simulink model "test_kalman_filter"  (R2020a)
settings: Solver=FixedStepAuto  StartTime=0.0  StopTime=85  RelTol=1e-3
values from neighbouring files (symbols this model uses):
  dt = 1/100    (= 0.01)    [load_tune.m]
  P0 = deg2rad(1)*eye(3,3)    [load_tune.m]
  Q = diag([a*pqr_dot_covar(1)*a /4, a*pqr_dot_covar(2)*a/4, a*pqr_dot_covar(3)*a/4])    [load_tune.m]
  R = diag([0.0155^2, 0.0124^2, 0.0147^2])    [load_tune.m]
  x0 = [0;0;0]    [load_tune.m]
undefined symbols (not defined in the file or in its folder): sim_data
libraries: myLib x3, simulink_extras x3, simulink x2, sharedtransform x1
settings Model: Creator=Test  LastModifiedBy=Jason
settings DataIOCC: ReturnWorkspaceOutputs=off
settings DebuggingCC: ArithmeticOperatorsInVariantConditions=warning
settings SFSimCC: SimUseLocalCustomCode=off  CustomCodeUndefinedFunction=UseInterfaceOnly
settings RTWCC: RTWUseLocalCustomCode=off

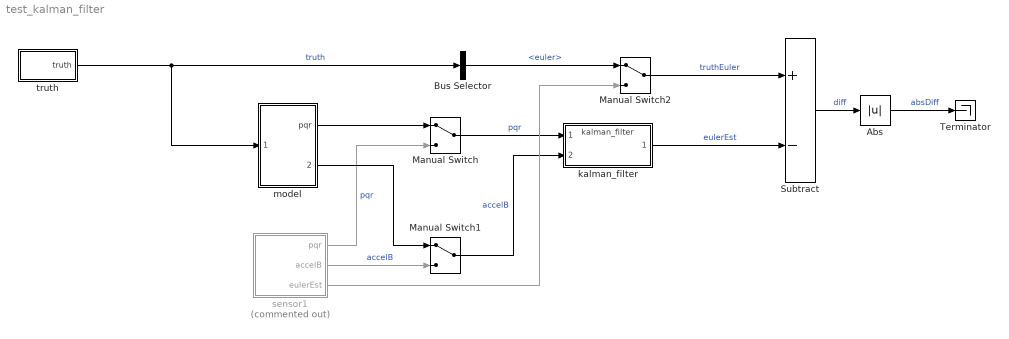
== system test_kalman_filter ==
  Abs : Abs
  Bus Selector : BusSelector  OutputSignals=euler
  Manual Switch : ManualSwitch
  Manual Switch1 : ManualSwitch
  Manual Switch2 : ManualSwitch
  Subtract : Sum  Inputs=+-
  Terminator : Terminator
  kalman_filter : ModelReference  ModelNameDialog=kalman_filter  ParameterArgumentNames=P0,Q,R,dt,x0  ParameterArgumentValues=P0,Q,R,dt,x0  UsingDefaultArgumentValue=0,0,0,0,0  SimulationMode=Normal  ModelReferenceVersion=1.264
  model : Subsystem  mask{SampleTime=dt}
      mask prompts: SampleTime "Simulink:blkprm_prompts:AllSrcBlksSampleTime"
      mask TypeOptions SampleTime:
      | Random
      | Number/SampleTime | Random
      | Number1/SampleTime | Zero-Order
      | Hold/SampleTime | Zero-Order
      | Hold1/SampleTime
      mask DialogControl SampleTime Prompt: Sample time:
  sensor1 : Subsystem  Commented=on  mask{SampleTime=dt}
      mask prompts: SampleTime "Simulink:blkprm_prompts:AllBlksSampleTime"
      mask TypeOptions SampleTime:
      | Zero-Order
      | Hold/SampleTime | Zero-Order
      | Hold1/SampleTime
      mask DialogControl SampleTime Prompt: Sample time (-1 for inherited):
  truth : Subsystem
  wires:
  Abs/1 -> Terminator/1  "absDiff"
  kalman_filter/1 -> Subtract/2  "eulerEst"
  truth/1(truth) -> model/1(truth), Bus Selector/1  "truth"
  Bus Selector/1 -> Manual Switch2/1  "<euler>"
  Manual Switch1/1 -> kalman_filter/2  "accelB"
  Manual Switch/1 -> kalman_filter/1  "pqr"
  Subtract/1 -> Abs/1  "diff"
  sensor1/2(accelB) -> Manual Switch1/2  "accelB"
  sensor1/1(pqr) -> Manual Switch/2  "pqr"
  model/2(accelB) -> Manual Switch1/1
  Manual Switch2/1 -> Subtract/1  "truthEuler"
  sensor1/3(eulerEst) -> Manual Switch2/2
  model/1(pqr) -> Manual Switch/1

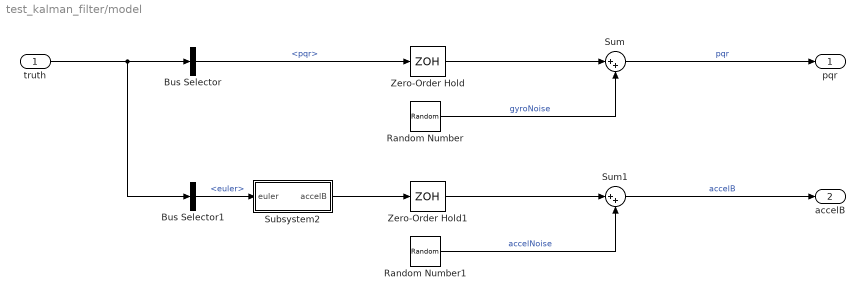
== system test_kalman_filter/model ==
  truth : Inport
  Bus Selector : BusSelector  OutputSignals=pqr
  Bus Selector1 : BusSelector  OutputSignals=euler
  Random Number : RandomNumber  Mean=sim_data.gyro.bias  Variance=sim_data.gyro.var  Seed=sim_data.gyro.seed  SampleTime=SampleTime
  Random Number1 : RandomNumber  Mean=sim_data.accel.bias  Variance=sim_data.accel.var  Seed=sim_data.accel.seed  SampleTime=SampleTime
  Subsystem2 : Subsystem
  Sum : Sum  Inputs=|++
  Sum1 : Sum  Inputs=|++
  Zero-Order Hold : ZeroOrderHold  SampleTime=SampleTime
  Zero-Order Hold1 : ZeroOrderHold  SampleTime=SampleTime
  pqr : Outport  VectorParamsAs1DForOutWhenUnconnected=off
  accelB : Outport  Port=2  VectorParamsAs1DForOutWhenUnconnected=off
  wires:
  truth/1 -> Bus Selector1/1, Bus Selector/1
  Random Number/1 -> Sum/2  "gyroNoise"
  Random Number1/1 -> Sum1/2  "accelNoise"
  Subsystem2/1(accelB) -> Zero-Order Hold1/1
  Bus Selector/1 -> Zero-Order Hold/1  "<pqr>"
  Bus Selector1/1 -> Subsystem2/1(euler)  "<euler>"
  Sum1/1 -> accelB/1  "accelB"
  Sum/1 -> pqr/1  "pqr"
  Zero-Order Hold/1 -> Sum/1
  Zero-Order Hold1/1 -> Sum1/1

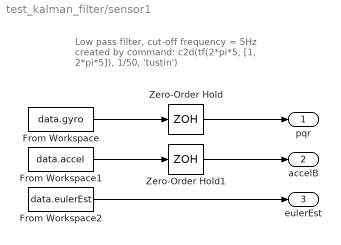
== system test_kalman_filter/sensor1 ==
  note: Low pass filter, cut-off frequency = 5Hz
      |
      | created by command:
      | c2d(tf(2*pi*5, [1, 2*pi*5]), 1/50, 'tustin')
  From Workspace : FromWorkspace  VariableName=data.gyro  OutputAfterFinalValue=Setting to zero
  From Workspace1 : FromWorkspace  VariableName=data.accel  OutputAfterFinalValue=Setting to zero
  From Workspace2 : FromWorkspace  VariableName=data.eulerEst  OutputAfterFinalValue=Setting to zero
  Zero-Order Hold : ZeroOrderHold  SampleTime=SampleTime
  Zero-Order Hold1 : ZeroOrderHold  SampleTime=SampleTime
  pqr : Outport  VectorParamsAs1DForOutWhenUnconnected=off
  accelB : Outport  Port=2  VectorParamsAs1DForOutWhenUnconnected=off
  eulerEst : Outport  Port=3  VectorParamsAs1DForOutWhenUnconnected=off
  wires:
  From Workspace/1 -> Zero-Order Hold/1
  From Workspace1/1 -> Zero-Order Hold1/1
  Zero-Order Hold/1 -> pqr/1
  Zero-Order Hold1/1 -> accelB/1
  From Workspace2/1 -> eulerEst/1

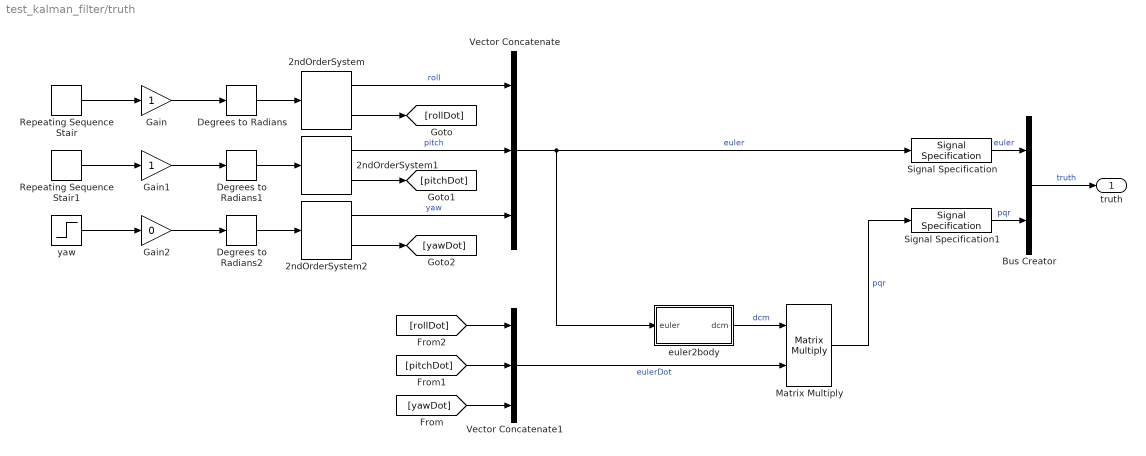
== system test_kalman_filter/truth ==
  2ndOrderSystem : myLib/2ndOrderSystem  wn=1  zeta=0.707  p0=sim_data.x0(1)  v0=0
  2ndOrderSystem1 : myLib/2ndOrderSystem  wn=1  zeta=0.707  p0=sim_data.x0(2)  v0=0
  2ndOrderSystem2 : myLib/2ndOrderSystem  wn=1  zeta=0.707  p0=sim_data.x0(3)  v0=0
  Bus Creator : BusCreator  Inputs=2
  Degrees to Radians : simulink_extras/Transformations/Degrees to Radians
  Degrees to Radians1 : simulink_extras/Transformations/Degrees to Radians
  Degrees to Radians2 : simulink_extras/Transformations/Degrees to Radians
  Gain : Gain
  Gain1 : Gain
  Gain2 : Gain  Gain=0
  Matrix Multiply : Product  Multiplication=Matrix(*)
  Repeating Sequence Stair : simulink/Sources/Repeating Sequence Stair  OutValues=[-10 10 45 30].'  tsamp=5  OutMin=[]  OutMax=[]  OutDataTypeStr=double  OutputDataTypeScalingMode=double  OutDataType=fixdt(0,8)  ConRadixGroup=Best Precision: Vector-wise  OutScaling=2^-12
      settings: AttributesFormatString=Ts = %<tsamp>s
  Repeating Sequence Stair1 : simulink/Sources/Repeating Sequence Stair  OutValues=[20 5 -10].'  tsamp=20  OutMin=[]  OutMax=[]  OutDataTypeStr=double  OutputDataTypeScalingMode=double  OutDataType=fixdt(0,8)  ConRadixGroup=Best Precision: Vector-wise  OutScaling=2^-12
      settings: AttributesFormatString=Ts = %<tsamp>s
  Signal Specification : SignalSpecification  Unit=rad  Dimensions=3
  Signal Specification1 : SignalSpecification  Unit=rad/s  Dimensions=3
  Vector Concatenate : Concatenate  NumInputs=3
  Vector Concatenate1 : Concatenate  NumInputs=3
  euler2body : MATLAB Function  TreatAsAtomicUnit=on
  yaw : Step  SampleTime=0
  truth : Outport  VectorParamsAs1DForOutWhenUnconnected=off
  wires:
  Degrees to Radians/1 -> 2ndOrderSystem/1
  Degrees to Radians1/1 -> 2ndOrderSystem1/1
  2ndOrderSystem2/1 -> Vector Concatenate/3  "yaw"
  2ndOrderSystem1/1 -> Vector Concatenate/2  "pitch"
  Degrees to Radians2/1 -> 2ndOrderSystem2/1
  yaw/1 -> Gain2/1
  2ndOrderSystem/1 -> Vector Concatenate/1  "roll"
  Vector Concatenate/1 -> euler2body/1(euler), Signal Specification/1  "euler"
  Bus Creator/1 -> truth/1  "truth"
  2ndOrderSystem/2 -> [rollDot]
  2ndOrderSystem1/2 -> [pitchDot]
  2ndOrderSystem2/2 -> [yawDot]
  [pitchDot] -> Vector Concatenate1/2
  [rollDot] -> Vector Concatenate1/1
  [yawDot] -> Vector Concatenate1/3
  Vector Concatenate1/1 -> Matrix Multiply/2  "eulerDot"
  Matrix Multiply/1 -> Signal Specification1/1  "pqr"
  euler2body/1(dcm) -> Matrix Multiply/1  "dcm"
  Signal Specification/1 -> Bus Creator/1  "euler"
  Signal Specification1/1 -> Bus Creator/2  "pqr"
  Gain/1 -> Degrees to Radians/1
  Gain1/1 -> Degrees to Radians1/1
  Gain2/1 -> Degrees to Radians2/1
  Repeating Sequence Stair/1 -> Gain/1
  Repeating Sequence Stair1/1 -> Gain1/1

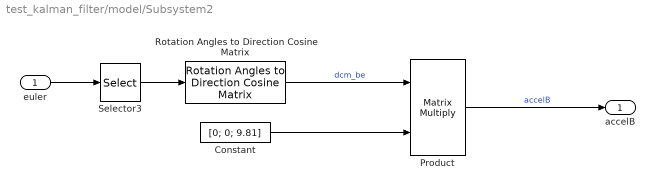
== system test_kalman_filter/model/Subsystem2 ==
  euler : Inport
  Constant : Constant  Value=[0; 0; 9.81]
  Product : Product  Multiplication=Matrix(*)
  Rotation Angles to Direction Cosine Matrix : sharedtransform/Rotation Angles to Direction Cosine Matrix  rotationOrder=ZYX  aMode=aMode
      settings: SourceProductBaseCode=AE,PW,MT,VE,VP
  Selector3 : Selector  InputPortWidth=3  IndexOptions=Index vector (dialog)  Indices=[3 2 1]  OutputSizes=1
  accelB : Outport  VectorParamsAs1DForOutWhenUnconnected=off
  wires:
  euler/1 -> Selector3/1
  Rotation Angles to Direction Cosine Matrix/1 -> Product/1  "dcm_be"
  Product/1 -> accelB/1  "accelB"
  Constant/1 -> Product/2
  Selector3/1 -> Rotation Angles to Direction Cosine Matrix/1

== matlab function test_kalman_filter/truth/euler2body ==
  data: dcm output; euler input
function dcm = fcn(euler)

phi = euler(1);
theta = euler(2);

% body to euler
% dcm = [
%     1 sin(phi)*tan(theta) cos(phi)*tan(theta);
%     0 cos(phi) -sin(phi);
%     0 sin(phi)*sec(theta) cos(phi)*sec(theta)];

% euler to body
dcm = [
    1 0 -sin(theta);
    0 cos(phi) sin(phi)*cos(theta);
    0 -sin(phi) cos(phi)*cos(theta)];

end
